simulink model "gm_uz_ninephase_VSD_transformation"  (R2021b)
settings: Solver=FixedStepAuto  StartTime=0.0  StopTime=inf  RelTol=1e-3
undefined symbols (not defined in the file or in its folder): a, b, c
libraries: hdlsllib x90, simulink x32, hdlmdlgenlib x20, dspsigops x7
(part 1 of 6)
settings Model: Creator=ts  LastModifiedBy=valen
settings SolverCC: AlgebraicLoopSolver=TrustRegion  AutoInsertRateTranBlk=on
settings DataIOCC: LimitDataPoints=on  SaveOutput=off  SaveTime=off
settings OptimizationCC: BlockReduction=off  ConditionallyExecuteInputs=off  DefaultParameterBehavior=Inlined  InheritOutputTypeSmallerThanSingle=on  LifeSpan=inf
settings DebuggingCC: AlgebraicLoopMsg=error  ArtificialAlgebraicLoopMsg=none  InheritedTsInSrcMsg=none  SingleTaskRateTransMsg=error  AllowSymbolicDim=off  StrictBusMsg=ErrorOnBusTreatedAsVector  SFUnexpectedBacktrackingDiag=warning  SFNoUnconditionalDefaultTransitionDiag=warning  SFExecutionAtInitializationDiag=none  SFMachineParentedDataDiag=warning  ArithmeticOperatorsInVariantConditions=warning
settings HardwareCC: ProdBitPerPointer=32  ProdBitPerSizeT=32  ProdBitPerPtrDiffT=32  ProdLargestAtomicFloat=None  ProdIntDivRoundTo=Undefined  ProdEndianess=Unspecified  ProdWordSize=32  ProdHWDeviceType=ASIC/FPGA->ASIC/FPGA  ProdEqTarget=off
settings SFSimCC: SimUseLocalCustomCode=off  CustomCodeUndefinedFunction=UseInterfaceOnly
settings RTWCC: RTWUseLocalCustomCode=off
settings CodeAppCC: StateflowObjectComments=on
settings GRTTargetCC: TargetLangStandard=C89/C90 (ANSI)
settings ConfigComp: CovScope=ReferencedModels  CovMetricSettings=dw  CovSaveCumulativeToWorkspaceVar=on  CovSaveSingleToWorkspaceVar=on  CovExternalEMLEnable=off  CovSFcnEnable=off

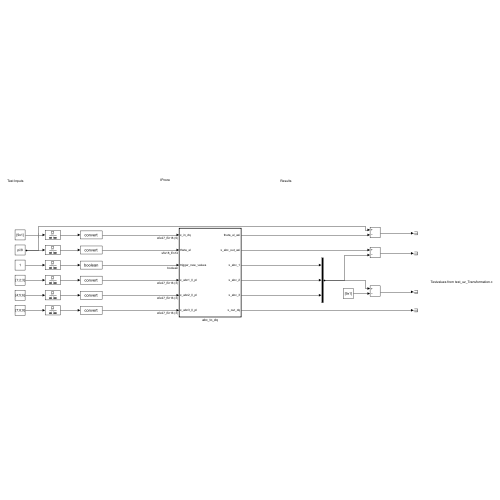
[thumbnail: Simulink's stored preview of the top-level diagram]
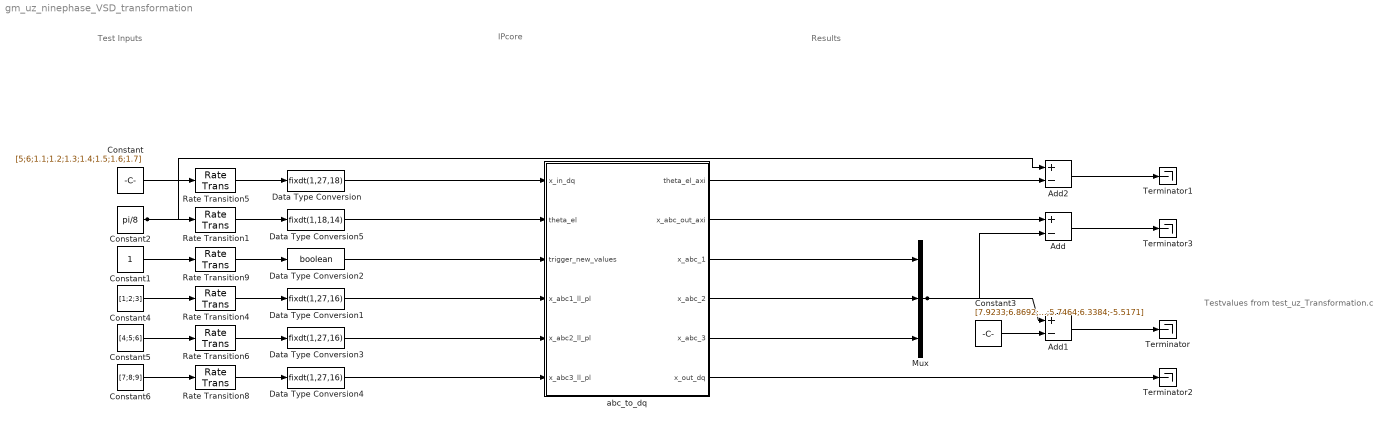
== system gm_uz_ninephase_VSD_transformation ==
  note: Testvalues from test_uz_Transformation.c
  note: IPcore
  note: Test Inputs
  note: Results
  Add : Sum  Inputs=+-
  Add1 : Sum  Inputs=+-
  Add2 : Sum  Inputs=+-
  Constant : Constant  Value=[5;6;1.1;1.2;1.3;1.4;1.5;1.6;1.7]
  Constant1 : Constant
  Constant2 : Constant  Value=pi/8
  Constant3 : Constant  Value=[7.9233;6.8692;-6.3925;5.6551;1.8092;-7.7966;5.7464;6.3384;-5.5171]  OutDataTypeStr=single
  Constant4 : Constant  Value=[1;2;3]
  Constant5 : Constant  Value=[4;5;6]
  Constant6 : Constant  Value=[7;8;9]
  Data Type Conversion : DataTypeConversion  OutDataTypeStr=fixdt(1,27,18)
  Data Type Conversion1 : DataTypeConversion  OutDataTypeStr=fixdt(1,27,16)
  Data Type Conversion2 : DataTypeConversion  OutDataTypeStr=boolean
  Data Type Conversion3 : DataTypeConversion  OutDataTypeStr=fixdt(1,27,16)
  Data Type Conversion4 : DataTypeConversion  OutDataTypeStr=fixdt(1,27,16)
  Data Type Conversion5 : DataTypeConversion  OutDataTypeStr=fixdt(1,18,14)
  Mux : Mux  Inputs=3
  Rate Transition{1,4..6,8..9} (6 alike) : RateTransition  OutPortSampleTime=ts_uz_ninephase_VSD_transformation
  Terminator{,1..3} (4 alike) : Terminator
  abc_to_dq : Subsystem  TreatAsAtomicUnit=on
  wires:
  Add/1 -> Terminator3/1
  Constant5/1 -> Rate Transition6/1
  Constant6/1 -> Rate Transition8/1
  Constant4/1 -> Rate Transition4/1
  abc_to_dq/6(x_out_dq) -> Terminator2/1
  Add2/1 -> Terminator1/1
  abc_to_dq/1(theta_el_axi) -> Add2/2
  Add1/1 -> Terminator/1
  Constant3/1 -> Add1/2
  abc_to_dq/2(x_abc_out_axi) -> Add/1
  Mux/1 -> Add/2, Add1/1
  abc_to_dq/4(x_abc_2) -> Mux/2
  abc_to_dq/5(x_abc_3) -> Mux/3
  abc_to_dq/3(x_abc_1) -> Mux/1
  Constant2/1 -> Rate Transition1/1, Add2/1
  Constant/1 -> Rate Transition5/1
  Rate Transition1/1 -> Data Type Conversion5/1
  Data Type Conversion5/1 -> abc_to_dq/2(theta_el)
  Constant1/1 -> Rate Transition9/1
  Rate Transition9/1 -> Data Type Conversion2/1
  Data Type Conversion2/1 -> abc_to_dq/3(trigger_new_values)
  Rate Transition8/1 -> Data Type Conversion4/1
  Rate Transition6/1 -> Data Type Conversion3/1
  Rate Transition4/1 -> Data Type Conversion1/1
  Data Type Conversion3/1 -> abc_to_dq/5(x_abc2_ll_pl)
  Data Type Conversion4/1 -> abc_to_dq/6(x_abc3_ll_pl)
  Rate Transition5/1 -> Data Type Conversion/1
  Data Type Conversion1/1 -> abc_to_dq/4(x_abc1_ll_pl)
  Data Type Conversion/1 -> abc_to_dq/1(x_in_dq)
